simulink model "bloc_filtru"  (R2017b)
settings: Solver=VariableStepAuto  StartTime=0.0  StopTime=10.0  RelTol=1e-3
settings Model: Creator=alinvoicu26  LastModifiedBy=alinvoicu26

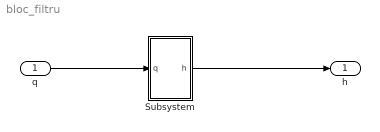
== system bloc_filtru ==
  "q " : Inport
  Subsystem : Subsystem
  "h " : Outport
  wires:
  "q "/1 -> Subsystem/1("q ")
  Subsystem/1("h ") -> "h "/1

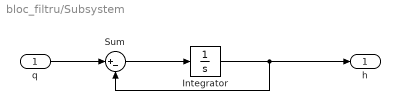
== system bloc_filtru/Subsystem ==
  "q " : Inport
  Integrator : Integrator
  Sum : Sum  Inputs=|+-
  "h " : Outport
  wires:
  Sum/1 -> Integrator/1
  "q "/1 -> Sum/1
  Integrator/1 -> "h "/1, Sum/2
